simulink model "rocket_ctrl"  (R2024b)
settings: Solver=VariableStepAuto  StartTime=0.0  StopTime=1.7  RelTol=1e-3
libraries: slpidlib x2, simulink_extras x2
settings Model: Creator=keybo  LastModifiedBy=keybo

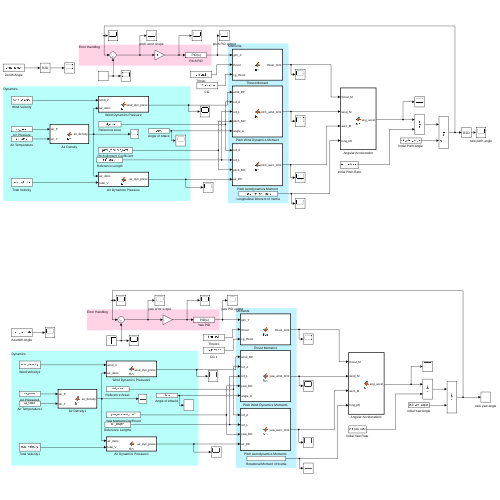
[thumbnail: Simulink's stored preview of the top-level diagram]
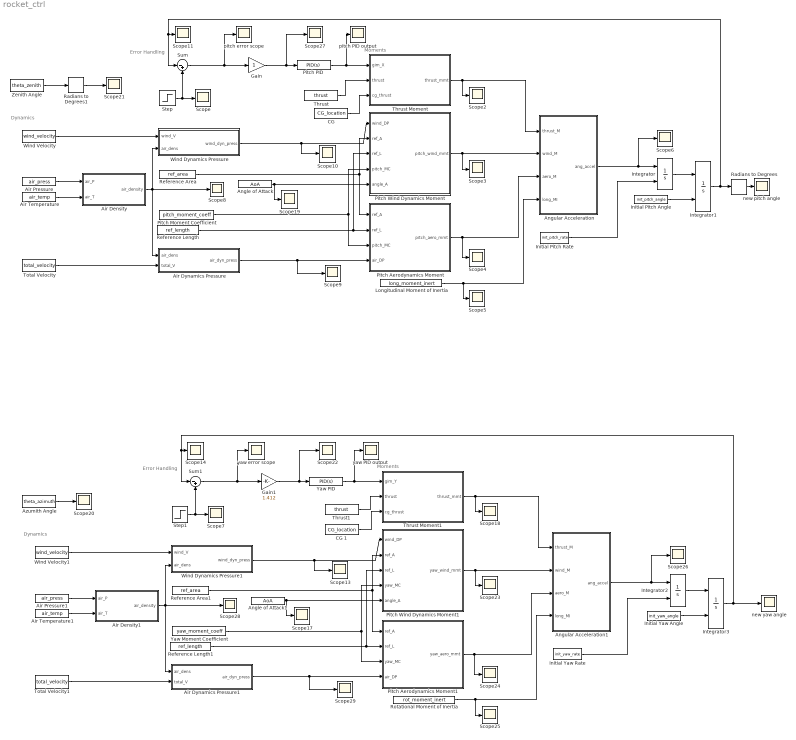
== system rocket_ctrl ==
  note: Error Handling
  note: Moments
  note: Dynamics
  note: Error Handling
  note: Dynamics
  note: Moments
  Air Density : MATLAB Function  TreatAsAtomicUnit=on
  Air Density1 : MATLAB Function  TreatAsAtomicUnit=on
  Air Dynamics Pressure : MATLAB Function  TreatAsAtomicUnit=on
  Air Dynamics Pressure1 : MATLAB Function  TreatAsAtomicUnit=on
  Air Pressure : FromWorkspace  VariableName=air_press
  Air Pressure1 : FromWorkspace  VariableName=air_press
  Air Temperature : FromWorkspace  VariableName=air_temp
  Air Temperature1 : FromWorkspace  VariableName=air_temp
  Angle of Attack : FromWorkspace  VariableName=AoA
  Angle of Attack1 : FromWorkspace  VariableName=AoA
  Angular Acceleration : MATLAB Function  TreatAsAtomicUnit=on
  Angular Acceleration1 : MATLAB Function  TreatAsAtomicUnit=on
  Azumith Angle : FromWorkspace  VariableName=theta_azimuth
  "CG " : FromWorkspace  VariableName=CG_location
  CG 1 : FromWorkspace  VariableName=CG_location
  Gain : Gain
  Gain1 : Gain  Gain=1.412
  Initial Pitch Angle : FromWorkspace  VariableName=init_pitch_angle
  Initial Pitch Rate : FromWorkspace  VariableName=init_pitch_rate
  Initial Yaw Angle : FromWorkspace  VariableName=init_yaw_angle
  Initial Yaw Rate : FromWorkspace  VariableName=init_yaw_rate
  Integrator{,1..3} (4 alike) : Integrator  InitialConditionSource=external
  Longitudinal Moment of Inertia : FromWorkspace  VariableName=long_moment_inert
  Pitch Aerodynamics Moment : MATLAB Function  TreatAsAtomicUnit=on
  Pitch Aerodynamics Moment1 : MATLAB Function  TreatAsAtomicUnit=on
  Pitch Moment Coefficient : FromWorkspace  VariableName=pitch_moment_coeff
  Pitch PID : slpidlib/PID Controller  Controller=PID  Form=Parallel  TimeDomain=Continuous-time  UseExternalTs=off  SampleTime=0.01  IntegratorMethod=Forward Euler  FilterMethod=Forward Euler  ControllerParametersSource=internal  P=0.297  I=0.00155  UseKiTs=off  D=0.0569  UseExternalDerivativeSource=off  N=20  UseFilter=on  TunerSelectOption=Transfer Function Based (PID Tuner App)  InitialConditionSource=internal  InitialConditionForIntegrator=0  InitialConditionForFilter=0  DifferentiatorICPrevScaledInput=0  ExternalReset=none  TrackingMode=off  Kt=1  LimitOutput=off  SatLimitsSource=internal  UpperSaturationLimit=0.1  LowerSaturationLimit=-0.5  LinearizeAsGain=off  AntiWindupMode=clamping  Kb=1  LimitIntegrator=off  UpperIntegratorSaturationLimit=0.5  LowerIntegratorSaturationLimit=-1  POutMin=[]  POutMax=[]  IOutMin=[]  IOutMax=[]  DOutMin=[]  DOutMax=[]  NOutMin=[]  NOutMax=[]  SumOutMin=[]  SumOutMax=[]  SaturationOutMin=[]  SaturationOutMax=[]  PParamMin=[]  PParamMax=[]  IParamMin=[]  IParamMax=[]  DParamMin=[]  DParamMax=[]  NParamMin=[]  NParamMax=[]  KbParamMin=[]  KbParamMax=[]  KtParamMin=[]  KtParamMax=[]  KbOutMin=[]  KbOutMax=[]  KtOutMin=[]  KtOutMax=[]  IntegratorOutMin=[]  IntegratorOutMax=[]  FilterOutMin=[]  FilterOutMax=[]  SumI1OutMin=[]  SumI1OutMax=[]  SumI2OutMin=[]  SumI2OutMax=[]  SumI3OutMin=[]  SumI3OutMax=[]  SumI4OutMin=[]  SumI4OutMax=[]  SumDOutMin=[]  SumDOutMax=[]  DifferentiatorOutMin=[]  DifferentiatorOutMax=[]  FilterDiffOutCoefMin=[]  FilterDiffOutCoefMax=[]  ReciprocalOutMin=[]  ReciprocalOutMax=[]  SumDenOutMin=[]  SumDenOutMax=[]  SumNumOutMin=[]  SumNumOutMax=[]  DivideOutMin=[]  DivideOutMax=[]  UdiffTsProdOutMin=[]  UdiffTsProdOutMax=[]  NTsProdOutMin=[]  NTsProdOutMax=[]  UintegralTsProdOutMin=[]  UintegralTsProdOutMax=[]  UngainTsProdOutMin=[]  UngainTsProdOutMax=[]  ClampingZeroOutDataTypeStr=Inherit: Inherit via back propagation  ClampingZeroOutMin=[]  ClampingZeroOutMax=[]  FilterDenConstantOutDataTypeStr=Inherit: Inherit via back propagation  FilterDenConstantOutMin=[]  FilterDenConstantOutMax=[]  PCopyOutDataTypeStr=Inherit: Inherit via back propagation  PCopyOutMin=[]  PCopyOutMax=[]  NCopyOutDataTypeStr=Inherit: Inherit via back propagation  NCopyOutMin=[]  NCopyOutMax=[]  IntegratorContinuousStateAttributes=''  IntegratorStateMustResolveToSignalObject=off  IntegratorRTWStateStorageClass=Auto  FilterContinuousStateAttributes=''  FilterStateMustResolveToSignalObject=off  FilterRTWStateStorageClass=Auto  ParallelPVariant=InternalParameters  IdealPVariant=Disabled  IVariant=InternalParameters  DVariant=InternalParameters  IntegratorVariant=Continuous  SatVariant=Disabled  AWVariant=Passthrough  PCopyVariant=Disabled  TRVariant=Disabled  FdbkBlocksVariant=Forward  IdealPFdbkVariant=Disabled  SatFdbkVariant=Disabled  DerivativeFilterVariant=ContFilter  NVariant=InternalParameters  NCopyVariant=Disabled  FilterICVariant=InternalICsFilter  IntegratorICVariant=InternalICs  ExternalResetVariant=Disabled  TRSumVariant=Passthrough  SumFdbkVariant=Disabled  SumVariant=Sum_PID  TsampFilterVariant=InternalTs  TsampNgainVariant=Passthrough  TsampIntegralVariant=Disabled_SignalSpec  ExternalSaturationOutDataTypeStr=Inherit: Same as second input  DerivativeSourceVariant=ErrorSignal  PreIntVariant=InternalPreInt
  Pitch Wind Dynamics Moment : MATLAB Function  TreatAsAtomicUnit=on
  Pitch Wind Dynamics Moment1 : MATLAB Function  TreatAsAtomicUnit=on
  Radians to Degrees : simulink_extras/Transformations/Radians to Degrees
  Radians to Degrees1 : simulink_extras/Transformations/Radians to Degrees
  Reference Area : FromWorkspace  VariableName=ref_area
  Reference Area1 : FromWorkspace  VariableName=ref_area
  Reference Length : FromWorkspace  VariableName=ref_length
  Reference Length1 : FromWorkspace  VariableName=ref_length
  Rotational Moment of Inertia : FromWorkspace  VariableName=rot_moment_inert
  Scope{,2..11,13..14,17..29} (26 alike) : Scope
  Step : Step  Time=0  After=0  SampleTime=0
  Step1 : Step  Time=0  After=0  SampleTime=0
  Sum : Sum  Inputs=|-+
  Sum1 : Sum  Inputs=|-+
  Thrust : FromWorkspace  VariableName=thrust
  Thrust Moment : MATLAB Function  TreatAsAtomicUnit=on
  Thrust Moment1 : MATLAB Function  TreatAsAtomicUnit=on
  Thrust1 : FromWorkspace  VariableName=thrust
  Total Velocity : FromWorkspace  VariableName=total_velocity
  Total Velocity1 : FromWorkspace  VariableName=total_velocity
  Wind Dynamics Pressure : MATLAB Function  TreatAsAtomicUnit=on
  Wind Dynamics Pressure1 : MATLAB Function  TreatAsAtomicUnit=on
  Wind Velocity : FromWorkspace  VariableName=wind_velocity
  Wind Velocity1 : FromWorkspace  VariableName=wind_velocity
  Yaw Moment Coefficient : FromWorkspace  VariableName=yaw_moment_coeff
  Yaw PID : slpidlib/PID Controller  Controller=PID  Form=Parallel  TimeDomain=Continuous-time  UseExternalTs=off  SampleTime=0.01  IntegratorMethod=Forward Euler  FilterMethod=Forward Euler  ControllerParametersSource=internal  P=0.00019838457011372  I=7.95594954545409e-05  UseKiTs=off  D=0.000120456605222877  UseExternalDerivativeSource=off  N=1142.8279760416  UseFilter=on  TunerSelectOption=Transfer Function Based (PID Tuner App)  InitialConditionSource=internal  InitialConditionForIntegrator=0  InitialConditionForFilter=0  DifferentiatorICPrevScaledInput=0  ExternalReset=none  TrackingMode=off  Kt=1  LimitOutput=off  SatLimitsSource=internal  UpperSaturationLimit=inf  LowerSaturationLimit=-inf  LinearizeAsGain=on  AntiWindupMode=none  Kb=1  LimitIntegrator=off  UpperIntegratorSaturationLimit=inf  LowerIntegratorSaturationLimit=-inf  POutMin=[]  POutMax=[]  IOutMin=[]  IOutMax=[]  DOutMin=[]  DOutMax=[]  NOutMin=[]  NOutMax=[]  SumOutMin=[]  SumOutMax=[]  SaturationOutMin=[]  SaturationOutMax=[]  PParamMin=[]  PParamMax=[]  IParamMin=[]  IParamMax=[]  DParamMin=[]  DParamMax=[]  NParamMin=[]  NParamMax=[]  KbParamMin=[]  KbParamMax=[]  KtParamMin=[]  KtParamMax=[]  KbOutMin=[]  KbOutMax=[]  KtOutMin=[]  KtOutMax=[]  IntegratorOutMin=[]  IntegratorOutMax=[]  FilterOutMin=[]  FilterOutMax=[]  SumI1OutMin=[]  SumI1OutMax=[]  SumI2OutMin=[]  SumI2OutMax=[]  SumI3OutMin=[]  SumI3OutMax=[]  SumI4OutMin=[]  SumI4OutMax=[]  SumDOutMin=[]  SumDOutMax=[]  DifferentiatorOutMin=[]  DifferentiatorOutMax=[]  FilterDiffOutCoefMin=[]  FilterDiffOutCoefMax=[]  ReciprocalOutMin=[]  ReciprocalOutMax=[]  SumDenOutMin=[]  SumDenOutMax=[]  SumNumOutMin=[]  SumNumOutMax=[]  DivideOutMin=[]  DivideOutMax=[]  UdiffTsProdOutMin=[]  UdiffTsProdOutMax=[]  NTsProdOutMin=[]  NTsProdOutMax=[]  UintegralTsProdOutMin=[]  UintegralTsProdOutMax=[]  UngainTsProdOutMin=[]  UngainTsProdOutMax=[]  ClampingZeroOutDataTypeStr=Inherit: Inherit via back propagation  ClampingZeroOutMin=[]  ClampingZeroOutMax=[]  FilterDenConstantOutDataTypeStr=Inherit: Inherit via back propagation  FilterDenConstantOutMin=[]  FilterDenConstantOutMax=[]  PCopyOutDataTypeStr=Inherit: Inherit via back propagation  PCopyOutMin=[]  PCopyOutMax=[]  NCopyOutDataTypeStr=Inherit: Inherit via back propagation  NCopyOutMin=[]  NCopyOutMax=[]  IntegratorContinuousStateAttributes=''  IntegratorStateMustResolveToSignalObject=off  IntegratorRTWStateStorageClass=Auto  FilterContinuousStateAttributes=''  FilterStateMustResolveToSignalObject=off  FilterRTWStateStorageClass=Auto  ParallelPVariant=InternalParameters  IdealPVariant=Disabled  IVariant=InternalParameters  DVariant=InternalParameters  IntegratorVariant=Continuous  SatVariant=Disabled  AWVariant=Passthrough  PCopyVariant=Disabled  TRVariant=Disabled  FdbkBlocksVariant=Forward  IdealPFdbkVariant=Disabled  SatFdbkVariant=Disabled  DerivativeFilterVariant=ContFilter  NVariant=InternalParameters  NCopyVariant=Disabled  FilterICVariant=InternalICsFilter  IntegratorICVariant=InternalICs  ExternalResetVariant=Disabled  TRSumVariant=Passthrough  SumFdbkVariant=Disabled  SumVariant=Sum_PID  TsampFilterVariant=InternalTs  TsampNgainVariant=Passthrough  TsampIntegralVariant=Disabled_SignalSpec  ExternalSaturationOutDataTypeStr=Inherit: Same as second input  DerivativeSourceVariant=ErrorSignal  PreIntVariant=InternalPreInt
  Zenith Angle : FromWorkspace  VariableName=theta_zenith
  new pitch angle : Scope
  new yaw angle : Scope
  pitch PID output : Scope
  pitch error scope : Scope
  yaw PID output : Scope
  yaw error scope : Scope
  wires:
  Air Temperature/1 -> Air Density/2(air_T)
  Air Pressure/1 -> Air Density/1(air_P)
  Air Density/1(air_density) -> Air Dynamics Pressure/1(air_dens), Scope8/1, Wind Dynamics Pressure/2(air_dens)
  Total Velocity/1 -> Air Dynamics Pressure/2(total_V)
  Wind Velocity/1 -> Wind Dynamics Pressure/1(wind_V)
  Reference Area/1 -> Pitch Wind Dynamics Moment/2(ref_A), Pitch Aerodynamics Moment/1(ref_A)
  Reference Length/1 -> Pitch Wind Dynamics Moment/3(ref_L), Pitch Aerodynamics Moment/2(ref_L)
  Wind Dynamics Pressure/1(wind_dyn_press) -> Pitch Wind Dynamics Moment/1(wind_DP), Scope10/1
  Pitch Moment Coefficient/1 -> Pitch Aerodynamics Moment/3(pitch_MC), Pitch Wind Dynamics Moment/4(pitch_MC)
  Air Dynamics Pressure/1(air_dyn_press) -> Scope9/1, Pitch Aerodynamics Moment/4(air_DP)
  "CG "/1 -> Thrust Moment/3(cg_thrust)
  Thrust/1 -> Thrust Moment/2(thrust)
  Thrust Moment/1(thrust_mmt) -> Angular Acceleration/1(thrust_M), Scope2/1
  Pitch Wind Dynamics Moment/1(pitch_wind_mmt) -> Scope3/1, Angular Acceleration/2(wind_M)
  Pitch Aerodynamics Moment/1(pitch_aero_mmt) -> Angular Acceleration/3(aero_M), Scope4/1
  Sum/1 -> Gain/1, pitch error scope/1
  Angle of Attack/1 -> Pitch Wind Dynamics Moment/5(angle_A), Scope19/1
  Step/1 -> Sum/2, Scope/1
  Initial Pitch Rate/1 -> Integrator/2
  Initial Pitch Angle/1 -> Integrator1/2
  Integrator1/1 -> Radians to Degrees/1, Scope11/1, Sum/1
  Integrator/1 -> Integrator1/1
  Zenith Angle/1 -> Radians to Degrees1/1
  Angular Acceleration/1(ang_accel) -> Scope6/1, Integrator/1
  Longitudinal Moment of Inertia/1 -> Angular Acceleration/4(long_MI), Scope5/1
  Gain/1 -> Scope27/1, Pitch PID/1
  Sum1/1 -> Gain1/1, yaw error scope/1
  Total Velocity1/1 -> Air Dynamics Pressure1/2(total_V)
  Angle of Attack1/1 -> Pitch Wind Dynamics Moment1/5(angle_A), Scope17/1
  Air Density1/1(air_density) -> Air Dynamics Pressure1/1(air_dens), Scope28/1, Wind Dynamics Pressure1/2(air_dens)
  Air Pressure1/1 -> Air Density1/1(air_P)
  Initial Yaw Angle/1 -> Integrator3/2
  Gain1/1 -> Scope22/1, Yaw PID/1
  Air Temperature1/1 -> Air Density1/2(air_T)
  Rotational Moment of Inertia/1 -> Angular Acceleration1/4(long_MI), Scope25/1
  Angular Acceleration1/1(ang_accel) -> Scope26/1, Integrator2/1
  Yaw PID/1 -> yaw PID output/1, Thrust Moment1/1(gim_Y)
  Azumith Angle/1 -> Scope20/1
  Thrust1/1 -> Thrust Moment1/2(thrust)
  Integrator2/1 -> Integrator3/1
  Air Dynamics Pressure1/1(air_dyn_press) -> Scope29/1, Pitch Aerodynamics Moment1/4(air_DP)
  Wind Dynamics Pressure1/1(wind_dyn_press) -> Pitch Wind Dynamics Moment1/1(wind_DP), Scope13/1
  CG 1/1 -> Thrust Moment1/3(cg_thrust)
  Thrust Moment1/1(thrust_mmt) -> Angular Acceleration1/1(thrust_M), Scope18/1
  Wind Velocity1/1 -> Wind Dynamics Pressure1/1(wind_V)
  Pitch Wind Dynamics Moment1/1(yaw_wind_mmt) -> Scope23/1, Angular Acceleration1/2(wind_M)
  Integrator3/1 -> new yaw angle/1, Scope14/1, Sum1/1
  Step1/1 -> Sum1/2, Scope7/1
  Pitch Aerodynamics Moment1/1(yaw_aero_mmt) -> Angular Acceleration1/3(aero_M), Scope24/1
  Reference Area1/1 -> Pitch Wind Dynamics Moment1/2(ref_A), Pitch Aerodynamics Moment1/1(ref_A)
  Reference Length1/1 -> Pitch Wind Dynamics Moment1/3(ref_L), Pitch Aerodynamics Moment1/2(ref_L)
  Yaw Moment Coefficient/1 -> Pitch Aerodynamics Moment1/3(yaw_MC), Pitch Wind Dynamics Moment1/4(yaw_MC)
  Initial Yaw Rate/1 -> Integrator2/2
  Pitch PID/1 -> pitch PID output/1, Thrust Moment/1(gim_X)
  Radians to Degrees/1 -> new pitch angle/1
  Radians to Degrees1/1 -> Scope21/1

== matlab function rocket_ctrl/Pitch Aerodynamics Moment1 ==
  data: ref_A input; yaw_aero_mmt output; ref_L input; yaw_MC input; air_DP input
function yaw_aero_mmt = fcn(ref_A, ref_L, yaw_MC, air_DP)
    yaw_aero_mmt = ref_L*ref_A*yaw_MC*air_DP;

== matlab function rocket_ctrl/Air Dynamics Pressure ==
  data: air_dens input; air_dyn_press output; total_V input
function air_dyn_press = fcn(air_dens, total_V)
    air_dyn_press = (air_dens*total_V^2)/2;

== matlab function rocket_ctrl/Pitch Wind Dynamics Moment1 ==
  data: wind_DP input; ref_A input; ref_L input; yaw_wind_mmt output; yaw_MC input; angle_A input
function yaw_wind_mmt = fcn(wind_DP, ref_A, ref_L, yaw_MC, angle_A)

    yaw_wind_mmt = ref_L*ref_A*wind_DP*yaw_MC*sin(angle_A);

== matlab function rocket_ctrl/Thrust Moment1 ==
  data: gim_Y input; thrust input; cg_thrust input; thrust_mmt output
function thrust_mmt = fcn(gim_Y, thrust, cg_thrust)
    thrust_mmt = thrust*cg_thrust*sin(gim_Y);

== matlab function rocket_ctrl/Wind Dynamics Pressure1 ==
  data: wind_V input; wind_dyn_press output; air_dens input
function wind_dyn_press = fcn(wind_V, air_dens)
    wind_dyn_press = (air_dens*wind_V^2)/2;

== matlab function rocket_ctrl/Air Density ==
  data: air_P input; air_density output; air_T input
function air_density = fcn(air_P, air_T)
    R = 287.05;
    air_density = air_P/(R*(air_T));

== matlab function rocket_ctrl/Wind Dynamics Pressure ==
  data: wind_V input; wind_dyn_press output; air_dens input
function wind_dyn_press = fcn(wind_V, air_dens)
    wind_dyn_press = (air_dens*wind_V^2)/2;

== matlab function rocket_ctrl/Pitch Wind Dynamics Moment ==
  data: wind_DP input; ref_A input; ref_L input; pitch_wind_mmt output; pitch_MC input; angle_A input
function pitch_wind_mmt = fcn(wind_DP, ref_A, ref_L, pitch_MC, angle_A)

    pitch_wind_mmt = ref_L*ref_A*wind_DP*pitch_MC*sin(angle_A);

== matlab function rocket_ctrl/Pitch Aerodynamics Moment ==
  data: ref_A input; pitch_aero_mmt output; ref_L input; pitch_MC input; air_DP input
function pitch_aero_mmt = fcn(ref_A, ref_L, pitch_MC, air_DP)
    pitch_aero_mmt = ref_L*ref_A*pitch_MC*air_DP;

== matlab function rocket_ctrl/Thrust Moment ==
  data: gim_X input; thrust input; cg_thrust input; thrust_mmt output
function thrust_mmt = fcn(gim_X, thrust, cg_thrust)
    thrust_mmt = thrust*cg_thrust*sin(gim_X);

== matlab function rocket_ctrl/Angular Acceleration ==
  data: thrust_M input; ang_accel output; wind_M input; aero_M input; long_MI input
function ang_accel = fcn(thrust_M, wind_M, aero_M, long_MI)
    ang_accel = (thrust_M+wind_M+aero_M)/long_MI;

== matlab function rocket_ctrl/Air Density1 ==
  data: air_P input; air_density output; air_T input
function air_density = fcn(air_P, air_T)
    R = 287.05;
    air_density = air_P/(R*(air_T));

== matlab function rocket_ctrl/Air Dynamics Pressure1 ==
  data: air_dens input; air_dyn_press output; total_V input
function air_dyn_press = fcn(air_dens, total_V)
    air_dyn_press = (air_dens*total_V^2)/2;

== matlab function rocket_ctrl/Angular Acceleration1 ==
  data: thrust_M input; ang_accel output; wind_M input; aero_M input; long_MI input
function ang_accel = fcn(thrust_M, wind_M, aero_M, long_MI)
    ang_accel = (thrust_M+wind_M+aero_M)/long_MI;
